simulink model "new_nncACCsystem_3_50"  (R2021a)
(part 4 of 8)

  "IW{2,1}(50,:)'" : Constant  Value=[0.09831930728921310647105968882897286675870418548583984375;-0.9004953846858345656301025883294641971588134765625;0.3823677520085151382289723187568597495555877685546875;0.2464552002173462097456280162077746354043483734130859375;-0.82699585891826610239974115756922401487827301025390625;0.95338104427702086152152105569257400929927825927734375;0.59983471601488458357920308117172680795192718505859375;-0.2431560155961964564408361866298946551978588104248046875;-0.4915589472905919077305725295445881783962249755859375;0.5604683311093250352996619767509400844573974609375;0.37246668189138087967648971243761479854583740234375;0.6904612206735942780966297505074180662631988525390625;0.92269362889317818599010934121906757354736328125;0.6827066130408410149499331964761950075626373291015625;-0.6024325902624660944439938248251564800739288330078125;-0.1302830293989370724627718800547881983220577239990234375;0.352554557373348398385815016808919608592987060546875;-0.8039137833628287044263061034143902361392974853515625;0.12884370512304454958751875892630778253078460693359375;-0.92962977011756553480381626286543905735015869140625;0.349019303662005675459312215025420300662517547607421875;0.46333545063241399208919801822048611938953399658203125;-0.5113190440235708678073933697305619716644287109375;-0.550160420252401305418743504560552537441253662109375;-0.884031633572082142791259684599936008453369140625;-0.5305330597791513280725439472007565200328826904296875;-0.651303613625856758773124965955503284931182861328125;-0.3304191802778431164000494391075335443019866943359375;-0.6321718696307974116876948755816556513309478759765625;0.9076759284686062301261699758470058441162109375;0.149012291778720662449586598086170852184295654296875;0.93981622205645454215527934138663113117218017578125;-0.74453875127945556844366592486039735376834869384765625;-0.7285135747479396517434224733733572065830230712890625;-0.59445864199330600285975378938019275665283203125;0.835818926478058887852284897235222160816192626953125;-0.0641762930311714219211438603451824747025966644287109375;-0.137130363488935425042569704601191915571689605712890625;-0.74833708243601815279788525003823451697826385498046875;-0.81460877139248299982909884420223534107208251953125;0.9507549549026756974257068577571772038936614990234375;-0.959279800618370703801929266774095594882965087890625;0.98522956213218382259810823597945272922515869140625;0.4539098666570862139479913821560330688953399658203125;0.8923848189255501051064811690594069659709930419921875;0.2144407114932208868740559637444675900042057037353515625;0.1963565203499378075679970834244159050285816192626953125;-0.69131103604621724212364597406121902167797088623046875;0.58317189573562144833118736642063595354557037353515625;0.229142953155083706207051363890059292316436767578125]
      mask Display: e = 0.06;c1 = [120 150 230]/255;c2 = ([120 150 230]+0)/383;c3 = ([120 150 230]+128)/383;patch([0 1 1 0],[0 0 1 1],c1);patch([0 1 1 1-e 1-e 0+e],[0 0 1 1-e 0+e 0+e],c2);patch([0 0 1 1-e 0+e 0+e],[0 1 1 1-e 1-e 0+e],c3);plot([0 1 1 0 0],[0 0 1 1 0]);disp('weights');
  "IW{2,1}(6,:)'" : Constant  Value=[-0.1329969518067103673164552901653223671019077301025390625;0.7585162910837504046668300361488945782184600830078125;0.9706399772185927421475071241729892790317535400390625;-0.308225663441152875066109118051826953887939453125;0.04743567448146883414050734018019284121692180633544921875;0.317797646048890103376294291592785157263278961181640625;0.89081475934814913220094467760645784437656402587890625;-0.6607282429186545069654812323278747498989105224609375;0.374086825560154323522255026546190492808818817138671875;0.940878582367052462842593740788288414478302001953125;-0.564082070424209103265411613392643630504608154296875;-0.5161234985242544315298118817736394703388214111328125;0.416953896319010974824692539186798967421054840087890625;-0.78046576273932810607902865740470588207244873046875;0.1470575919358021454996787724667228758335113525390625;-0.8651243900321985424994863933534361422061920166015625;-0.690342757578949584029714969801716506481170654296875;0.085644176430526020027400591061450541019439697265625;0.39524722600505179936902777626528404653072357177734375;-0.080628491560736481602589265094138681888580322265625;0.45013622063989799926275736652314662933349609375;0.7668144595271026986438300809822976589202880859375;0.9603057924449840410119350053719244897365570068359375;0.370986811718405196103276466601528227329254150390625;0.1915382316144444985184236429631710052490234375;-0.44516273255462290858730511899921111762523651123046875;0.07585867679898004867222738312193541787564754486083984375;0.6987626542530727125068779059802182018756866455078125;0.5927383397099081907555273573962040245532989501953125;-0.1484669031003333916629571831435896456241607666015625;-0.473944458016541059208748265518806874752044677734375;0.961571911925642286433912886423058807849884033203125;0.89710887685689311155101677286438643932342529296875;-0.806895836872141725137907997122965753078460693359375;-0.0616084532832805731317193931317888200283050537109375;0.1127111425186899662520545462029986083507537841796875;-0.0662465586388905902648360779494396410882472991943359375;-0.619333622031219999115592145244590938091278076171875;0.2110399520989479638100050351567915640771389007568359375;-0.04788964753628847936806067764337058179080486297607421875;0.3615037281565192106569384122849442064762115478515625;0.93017748101764430312954345936304889619350433349609375;-0.432877805142993121734207306872121989727020263671875;-0.509690606903658416371172279468737542629241943359375;0.952134378865099773037172781187109649181365966796875;-0.14222134871936542577230966344359330832958221435546875;-0.1188700564767217471295879249737481586635112762451171875;0.524936765335405564059101379825733602046966552734375;0.33819425820788440173458866411237977445125579833984375;0.5031966340243803070819694767124019563198089599609375]
      mask Display: e = 0.06;c1 = [120 150 230]/255;c2 = ([120 150 230]+0)/383;c3 = ([120 150 230]+128)/383;patch([0 1 1 0],[0 0 1 1],c1);patch([0 1 1 1-e 1-e 0+e],[0 0 1 1-e 0+e 0+e],c2);patch([0 0 1 1-e 0+e 0+e],[0 1 1 1-e 1-e 0+e],c3);plot([0 1 1 0 0],[0 0 1 1 0]);disp('weights');
  "IW{2,1}(7,:)'" : Constant  Value=[-0.378380611869383154388657430899911560118198394775390625;0.00914148396719571820767669123597443103790283203125;0.1067189467550966330833261963562108576297760009765625;0.953859982751964263769650642643682658672332763671875;0.26921353204869380437713743958738632500171661376953125;-0.466598925666688202351650716082076542079448699951171875;0.408076442193130051183658224545069970190525054931640625;0.353408168245023468490018103693728335201740264892578125;0.3648611927849430003334418870508670806884765625;-0.50809297008046272470238591267843730747699737548828125;-0.9606131086492462056725116781308315694332122802734375;-0.701854750336031951718496202374808490276336669921875;0.3850070775758960284207432778202928602695465087890625;0.3752484398438540313946987225790508091449737548828125;-0.4003218248306410487202811054885387420654296875;-0.79410834247234129978920691428356803953647613525390625;-0.79137545580738721806568491956568323075771331787109375;0.1333086108530838753694069964694790542125701904296875;-0.34363686854259345437867523287422955036163330078125;0.3759796645445596663392962000216357409954071044921875;-0.35483825434867366510616193409077823162078857421875;0.38348019107737696398174875866970978677272796630859375;0.107778350914894627265994131448678672313690185546875;-0.4597102130095780392338156161713413894176483154296875;-0.53141332210451175388499223117833025753498077392578125;-0.487841982872304458229706369820632971823215484619140625;-0.21919196467561119501255006980500183999538421630859375;-0.6621015042149169804730490795918740332126617431640625;0.593686659924843151969753307639621198177337646484375;0.8951819733576791282558815510128624737262725830078125;-0.8226175386358101082606708587263710796833038330078125;-0.0524424296605634499002235315856523811817169189453125;-0.287438490929447787447514883751864545047283172607421875;0.2568938160258849023875882267020642757415771484375;0.0234713512283253322721066069789230823516845703125;-0.52015759585506060602710931561887264251708984375;0.53486979578984150673903741335379891097545623779296875;0.5315809239871658320453207124955952167510986328125;0.09915883023369227722287888582286541350185871124267578125;0.38459946973296388339491613805876113474369049072265625;-0.2148888610536572318920889301807619631290435791015625;0.76280061728375425644799179281108081340789794921875;0.5352623766462112353536895170691423118114471435546875;0.047256088442521271275609251460991799831390380859375;0.2259328447102344483710112399421632289886474609375;0.388978386730647385238768265480757690966129302978515625;-0.409256795076363033558664028532803058624267578125;0.70697942760284371299661643206491135060787200927734375;-0.061122753349015158941259784342037164606153964996337890625;-0.9827527352508138580589047705871053040027618408203125]
      mask Display: e = 0.06;c1 = [120 150 230]/255;c2 = ([120 150 230]+0)/383;c3 = ([120 150 230]+128)/383;patch([0 1 1 0],[0 0 1 1],c1);patch([0 1 1 1-e 1-e 0+e],[0 0 1 1-e 0+e 0+e],c2);patch([0 0 1 1-e 0+e 0+e],[0 1 1 1-e 1-e 0+e],c3);plot([0 1 1 0 0],[0 0 1 1 0]);disp('weights');
  "IW{2,1}(8,:)'" : Constant  Value=[-0.0700909247488262499015121420598006807267665863037109375;0.0011918080437052225306615582667291164398193359375;-0.321425877976542206937438095337711274623870849609375;0.1797279974684445058574766562742297537624835968017578125;-0.61813010948421320822632196723134256899356842041015625;0.78385704015674095845866986564942635595798492431640625;0.8221964279291029686902447792817838490009307861328125;0.209828508283590842165011736142332665622234344482421875;0.6642603824305266524419266715995036065578460693359375;0.92725822907150445839619123944430612027645111083984375;0.3951073228096628753291952307336032390594482421875;0.262182553519213712434066110290586948394775390625;0.27733903857953701166394466781639494001865386962890625;0.5560488791469826441726809207466430962085723876953125;-0.5187997185350738948983462250907905399799346923828125;-0.341426288256590326763983966884552501142024993896484375;0.25149242499956414587103381563792936503887176513671875;0.755111935257769761875579206389375030994415283203125;-0.405882637490638964461453497278853319585323333740234375;0.9404243329614481172740170222823508083820343017578125;0.707661010677071544705540873110294342041015625;0.495089474961616426984534200528287328779697418212890625;0.013815382745125504015959450043737888336181640625;-0.11761351242806039607557977433316409587860107421875;-0.03481894705463643713283516945011797361075878143310546875;-0.21111948085500842342554506103624589741230010986328125;0.151995190502329791115698753856122493743896484375;0.8027562352749608720614560297690331935882568359375;0.8444176632681534844238058212795294821262359619140625;0.9360286508372592795268474219483323395252227783203125;-0.635066231519643142888753573060967028141021728515625;-0.193956021305207837457373898359946906566619873046875;-0.266720301626569511466158246548729948699474334716796875;0.008791188502246694014274908113293349742889404296875;0.649433339723579639013451014761812984943389892578125;0.9187562695995519224112513256841339170932769775390625;-0.457709580746702815456927737614023499190807342529296875;-0.7935593338441579991382468506344594061374664306640625;-0.87804597112296500771577711930149234831333160400390625;0.86494885279450806070400403768871910870075225830078125;0.6141326902204469195822866822709329426288604736328125;0.98700515167720814790897065904573537409305572509765625;-0.95134978734591790772157082756166346371173858642578125;0.231683711896522481765714474022388458251953125;0.5504355731980201671404984153923578560352325439453125;0.021550459646368584631925813255293178372085094451904296875;-0.1509322868245421556121499406799557618796825408935546875;0.80331171205689921865911173881613649427890777587890625;0.0647157520143744890983583673005341552197933197021484375;-0.92141740456274856541085682692937552928924560546875]
      mask Display: e = 0.06;c1 = [120 150 230]/255;c2 = ([120 150 230]+0)/383;c3 = ([120 150 230]+128)/383;patch([0 1 1 0],[0 0 1 1],c1);patch([0 1 1 1-e 1-e 0+e],[0 0 1 1-e 0+e 0+e],c2);patch([0 0 1 1-e 0+e 0+e],[0 1 1 1-e 1-e 0+e],c3);plot([0 1 1 0 0],[0 0 1 1 0]);disp('weights');
  "IW{2,1}(9,:)'" : Constant  Value=[-0.3375495316163341641413353499956429004669189453125;0.1207458837756620884107405800023116171360015869140625;-0.36098916461293395485654400545172393321990966796875;0.1811186112838754080911485289107076823711395263671875;0.308589790555177767572558877873234450817108154296875;-0.57997586211291274338464063475839793682098388671875;-0.7638434122699784278864854059065692126750946044921875;-0.969638202128953796687937938258983194828033447265625;-0.4858800234349580637882581868325360119342803955078125;0.465948763194291348810338604380376636981964111328125;0.284992410587107780628457476268522441387176513671875;0.0710664164131202813479148971964605152606964111328125;0.4275054573353702647153795624035410583019256591796875;-0.7260096518567333845339817344211041927337646484375;0.2765567368307468854027320048771798610687255859375;0.3561882324253777820644017992890439927577972412109375;-0.4205020372613805790251717553474009037017822265625;-0.8080969169396523543724697447032667696475982666015625;0.4349337843805700654087331713526509702205657958984375;0.1703146924140643836409481082228012382984161376953125;-0.7730840059185679624675913146347738802433013916015625;0.1869939554115604973816289202659390866756439208984375;0.7484598006972114081492009063367731869220733642578125;-0.71160521484614935872059504617936909198760986328125;0.3545085085218275811058674662490375339984893798828125;-0.4724444510508922778768692296580411493778228759765625;0.9443269128541891266337415800080634653568267822265625;-0.6033969317398566456489561460330151021480560302734375;0.2287814224476465430058169658877886831760406494140625;0.73622335616663736601594791864044964313507080078125;0.43880181030830467392434002249501645565032958984375;0.33867593506663684621571519528515636920928955078125;-0.911758023490152336165692759095691144466400146484375;-0.1675746774870845445803979600896127521991729736328125;-0.7491345627653753780350598390214145183563232421875;0.376110387437833093571271092514507472515106201171875;0.64029367354093924546987182111479341983795166015625;-0.68406754428360461162128558498807251453399658203125;-0.51146627236871200494761069421656429767608642578125;0.9035500291504694470035019548959098756313323974609375;-0.17041612963182917184212783467955887317657470703125;0.480264888283480129160807337029837071895599365234375;0.126183353962001643111534576746635138988494873046875;-0.9719103988274333527641601904178969562053680419921875;0.4723716954471957052419384126551449298858642578125;-0.9837458298014210011928071253350935876369476318359375;-0.4624498703158013146463645171024836599826812744140625;-0.7074306152282689996724229786195792257785797119140625;0.021891878844727319375351726193912327289581298828125;-0.5595792013797631359039996823412366211414337158203125]
      mask Display: e = 0.06;c1 = [120 150 230]/255;c2 = ([120 150 230]+0)/383;c3 = ([120 150 230]+128)/383;patch([0 1 1 0],[0 0 1 1],c1);patch([0 1 1 1-e 1-e 0+e],[0 0 1 1-e 0+e 0+e],c2);patch([0 0 1 1-e 0+e 0+e],[0 1 1 1-e 1-e 0+e],c3);plot([0 1 1 0 0],[0 0 1 1 0]);disp('weights');
  Mux : Mux  Inputs=50
      mask Display: e = 0.06;c1 = [120 150 230]/255;c2 = ([120 150 230]+0)/383;c3 = ([120 150 230]+128)/383;patch([0 1 1 0],[0 0 1 1],c1);patch([0 1 1 1-e 1-e 0+e],[0 0 1 1-e 0+e 0+e],c2);patch([0 0 1 1-e 0+e 0+e],[0 1 1 1-e 1-e 0+e],c3);plot([0 1 1 0 0],[0 0 1 1 0]);disp('Mux');
  dotprod{1..50} (50 alike) : neural/Weight Functions/dotprod
  "lz{2,1}" : Outport
      mask Display: e = 0.06;c1 = [120 230 180]/255;c2 = ([120 230 180]+0)/(256+128);c3 = ([120 230 180]+128)/(256+128);patch([0 1 1 0],[0 0 1 1],c1);patch([0 1 1 1-e 1-e 0+e],[0 0 1 1-e 0+e 0+e],c2);patch([0 0 1 1-e 0+e 0+e],[0 1 1 1-e 1-e 0+e],c3);plot([0 1 1 0 0],[0 0 1 1 0]);
  wires:
  "IW{2,1}(1,:)'"/1 -> dotprod1/1
  "ad{2,1}"/1 -> dotprod1/2, dotprod2/2, dotprod3/2, dotprod4/2, dotprod5/2, dotprod6/2, dotprod7/2, dotprod8/2, dotprod9/2, dotprod10/2, dotprod11/2, dotprod12/2, dotprod13/2, dotprod14/2, dotprod15/2, dotprod16/2, dotprod17/2, dotprod18/2, dotprod19/2, dotprod20/2, dotprod21/2, dotprod22/2, dotprod23/2, dotprod24/2, dotprod25/2, dotprod26/2, dotprod27/2, dotprod28/2, dotprod29/2, dotprod30/2, dotprod31/2, dotprod32/2, dotprod33/2, dotprod34/2, dotprod35/2, dotprod36/2, dotprod37/2, dotprod38/2, dotprod39/2, dotprod40/2, dotprod41/2, dotprod42/2, dotprod43/2, dotprod44/2, dotprod45/2, dotprod46/2, dotprod47/2, dotprod48/2, dotprod49/2, dotprod50/2
  dotprod1/1 -> Mux/1
  "IW{2,1}(2,:)'"/1 -> dotprod2/1
  dotprod2/1 -> Mux/2
  "IW{2,1}(3,:)'"/1 -> dotprod3/1
  dotprod3/1 -> Mux/3
  "IW{2,1}(4,:)'"/1 -> dotprod4/1
  dotprod4/1 -> Mux/4
  "IW{2,1}(5,:)'"/1 -> dotprod5/1
  dotprod5/1 -> Mux/5
  "IW{2,1}(6,:)'"/1 -> dotprod6/1
  dotprod6/1 -> Mux/6
  "IW{2,1}(7,:)'"/1 -> dotprod7/1
  dotprod7/1 -> Mux/7
  "IW{2,1}(8,:)'"/1 -> dotprod8/1
  dotprod8/1 -> Mux/8
  "IW{2,1}(9,:)'"/1 -> dotprod9/1
  dotprod9/1 -> Mux/9
  "IW{2,1}(10,:)'"/1 -> dotprod10/1
  dotprod10/1 -> Mux/10
  "IW{2,1}(11,:)'"/1 -> dotprod11/1
  dotprod11/1 -> Mux/11
  "IW{2,1}(12,:)'"/1 -> dotprod12/1
  dotprod12/1 -> Mux/12
  "IW{2,1}(13,:)'"/1 -> dotprod13/1
  dotprod13/1 -> Mux/13
  "IW{2,1}(14,:)'"/1 -> dotprod14/1
  dotprod14/1 -> Mux/14
  "IW{2,1}(15,:)'"/1 -> dotprod15/1
  dotprod15/1 -> Mux/15
  "IW{2,1}(16,:)'"/1 -> dotprod16/1
  dotprod16/1 -> Mux/16
  "IW{2,1}(17,:)'"/1 -> dotprod17/1
  dotprod17/1 -> Mux/17
  "IW{2,1}(18,:)'"/1 -> dotprod18/1
  dotprod18/1 -> Mux/18
  "IW{2,1}(19,:)'"/1 -> dotprod19/1
  dotprod19/1 -> Mux/19
  "IW{2,1}(20,:)'"/1 -> dotprod20/1
  dotprod20/1 -> Mux/20
  "IW{2,1}(21,:)'"/1 -> dotprod21/1
  dotprod21/1 -> Mux/21
  "IW{2,1}(22,:)'"/1 -> dotprod22/1
  dotprod22/1 -> Mux/22
  "IW{2,1}(23,:)'"/1 -> dotprod23/1
  dotprod23/1 -> Mux/23
  "IW{2,1}(24,:)'"/1 -> dotprod24/1
  dotprod24/1 -> Mux/24
  "IW{2,1}(25,:)'"/1 -> dotprod25/1
  dotprod25/1 -> Mux/25
  "IW{2,1}(26,:)'"/1 -> dotprod26/1
  dotprod26/1 -> Mux/26
  "IW{2,1}(27,:)'"/1 -> dotprod27/1
  dotprod27/1 -> Mux/27
  "IW{2,1}(28,:)'"/1 -> dotprod28/1
  dotprod28/1 -> Mux/28
  "IW{2,1}(29,:)'"/1 -> dotprod29/1
  dotprod29/1 -> Mux/29
  "IW{2,1}(30,:)'"/1 -> dotprod30/1
  dotprod30/1 -> Mux/30
  "IW{2,1}(31,:)'"/1 -> dotprod31/1
  dotprod31/1 -> Mux/31
  "IW{2,1}(32,:)'"/1 -> dotprod32/1
  dotprod32/1 -> Mux/32
  "IW{2,1}(33,:)'"/1 -> dotprod33/1
  dotprod33/1 -> Mux/33
  "IW{2,1}(34,:)'"/1 -> dotprod34/1
  dotprod34/1 -> Mux/34
  "IW{2,1}(35,:)'"/1 -> dotprod35/1
  dotprod35/1 -> Mux/35
  "IW{2,1}(36,:)'"/1 -> dotprod36/1
  dotprod36/1 -> Mux/36
  "IW{2,1}(37,:)'"/1 -> dotprod37/1
  dotprod37/1 -> Mux/37
  "IW{2,1}(38,:)'"/1 -> dotprod38/1
  dotprod38/1 -> Mux/38
  "IW{2,1}(39,:)'"/1 -> dotprod39/1
  dotprod39/1 -> Mux/39
  "IW{2,1}(40,:)'"/1 -> dotprod40/1
  dotprod40/1 -> Mux/40
  "IW{2,1}(41,:)'"/1 -> dotprod41/1
  dotprod41/1 -> Mux/41
  "IW{2,1}(42,:)'"/1 -> dotprod42/1
  dotprod42/1 -> Mux/42
  "IW{2,1}(43,:)'"/1 -> dotprod43/1
  dotprod43/1 -> Mux/43
  "IW{2,1}(44,:)'"/1 -> dotprod44/1
  dotprod44/1 -> Mux/44
  "IW{2,1}(45,:)'"/1 -> dotprod45/1
  dotprod45/1 -> Mux/45
  "IW{2,1}(46,:)'"/1 -> dotprod46/1
  dotprod46/1 -> Mux/46
  "IW{2,1}(47,:)'"/1 -> dotprod47/1
  dotprod47/1 -> Mux/47
  "IW{2,1}(48,:)'"/1 -> dotprod48/1
  dotprod48/1 -> Mux/48
  "IW{2,1}(49,:)'"/1 -> dotprod49/1
  dotprod49/1 -> Mux/49
  "IW{2,1}(50,:)'"/1 -> dotprod50/1
  dotprod50/1 -> Mux/50
  Mux/1 -> "lz{2,1}"/1
